simulink model "demo_gs2"  (Simulink 2.20)
settings: Solver=ode45  StartTime=0.0  StopTime=15  MaxStep=0.1  RelTol=1e-3  AbsTol=1e-6
values from neighbouring files (symbols this model uses):
  v = menu('EXACT LINEARIZATION (demo simulations)',    'Exact linearization of SISO system',    'Exact linearization of MIMO system',    'System with unstable zero dynamics')    [demos_exakt.m]    (also in demos_fp.m = menu('PHASE PLANE ANALYSIS (demo simulations)',    '2nd-Orde; demos_gs.m = menu('GAIN SCHEDULING (demo simulations)',    'Input and out)
  x1 = x(j)    [fazrov_auton2.m]
  x2 = x(j+1)    [fazrov_auton2.m]    (also in fazrov_typ1.m = get_param(get_param(gcbh,'Parent'),'UserData'))
undefined symbols (not defined in the file or in its folder): w
libraries: NelinSys x10
settings Model: ConsistencyChecking=off  RTWPlaceOutputsASAP=off

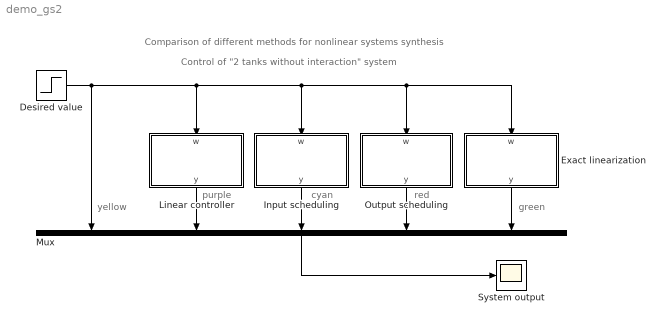
== system demo_gs2 ==
  note: Comparison of different methods for nonlinear systems synthesis
  note: Control of "2 tanks without interaction" system
  note: yellow
  note: purple
  note: cyan
  note: red
  note: green
  Desired value : Step  Time=5  Before=1  After=10
  Exact linearization : Subsystem  Orientation=down
      mask Type: Exact linearization
      mask Display: disp('Exact\nlinearization');
  Input scheduling : Subsystem  Orientation=down
      mask Type: Input scheduling
      mask Display: disp('Input\nscheduling');
  Linear controller : Subsystem  Orientation=down
      mask Type: Linear controller
      mask Display: disp('Linear\ncontroller');
  Mux : Mux  Orientation=down  Inputs=5
  Output scheduling : Subsystem  Orientation=down
      mask Type: Output scheduling
      mask Display: disp('Output\nscheduling');
  System output : Scope
      settings: TickLabels=on  TimeRange=15  YMin=0  YMax=12  SaveToWorkspace=off  SaveName=ScopeData
  wires:
  Output scheduling/1(y) -> Mux/4
  Input scheduling/1(y) -> Mux/3
  Linear controller/1(y) -> Mux/2
  Exact linearization/1(y) -> Mux/5
  Desired value/1 -> Mux/1, Linear controller/1(w), Input scheduling/1(w), Output scheduling/1(w), Exact linearization/1(w)
  Mux/1 -> System output/1

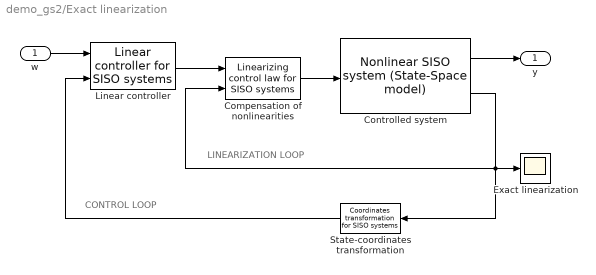
== system demo_gs2/Exact linearization ==
  note: LINEARIZATION LOOP
  note: CONTROL LOOP
  w : Inport  Port=1  PortWidth=-1  SampleTime=-1
  Compensation of nonlinearities : NelinSys/Nonlinear Systems Synthesis/Exact Linearization Blocks/Linearizing control law for SISO systems  n=2  vzorec=x1/sqrt(x2)+2*sqrt(x1)*v  vzorecP=0
  Controlled system : NelinSys/Nonlinear Systems Synthesis/Nonlinear SISO system (State-Space model)  n=2  F=[-sqrt(x1); sqrt(x1)-sqrt(x2)]  Fp=0  G=[1; 0]  Gp=0  H=x2  Hp=0  pp=[0.1; 0.01]
  Exact linearization : Scope
      settings: TickLabels=on  TimeRange=auto  YMin=0  YMax=12  SaveToWorkspace=off  SaveName=ScopeData
  Linear controller : NelinSys/Nonlinear Systems Synthesis/Exact Linearization Blocks/Linear controller for SISO systems  r=2  kor=[-2 -2]  integ=off
  State-coordinates transformation : NelinSys/Nonlinear Systems Synthesis/Exact Linearization Blocks/Coordinates transformation for SISO systems  Orientation=left  n=2  r=2  Z=[x2; sqrt(x1)-sqrt(x2)]  Zp=0
  y : Outport  Port=1
  wires:
  Compensation of nonlinearities/1 -> Controlled system/1
  Linear controller/1 -> Compensation of nonlinearities/1
  State-coordinates transformation/1 -> Linear controller/2
  Controlled system/2 -> State-coordinates transformation/1, Compensation of nonlinearities/2, Exact linearization/1
  w/1 -> Linear controller/1
  Controlled system/1 -> y/1

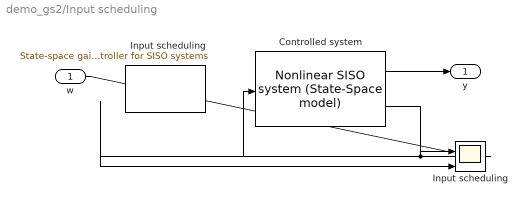
== system demo_gs2/Input scheduling ==
  w : Inport  Port=1  PortWidth=-1  SampleTime=-1
  Controlled system : NelinSys/Nonlinear Systems Synthesis/Nonlinear SISO system (State-Space model)  n=2  F=[-sqrt(x1); sqrt(x1)-sqrt(x2)]  Fp=0  G=[1; 0]  Gp=0  H=x2  Hp=0  pp=[0.1; 0.01]
  Input scheduling : Scope
      settings: TickLabels=on  TimeRange=auto  YMin=0  YMax=12  SaveToWorkspace=off  SaveName=ScopeData
  Input scheduling : NelinSys/Nonlinear Systems Synthesis/Gain Scheduling Blocks/State-space gain-scheduling controller for SISO systems  n=2  vzorec=-(-w^(1/2)+4*w)/w*x1+4*w+1/2*(-w^(1/2)+8*w-16*w^(3/2))/w*(x2-w)  vzorecP=0
  y : Outport  Port=1
  wires:
  Input scheduling/1 -> Controlled system/1
  Controlled system/2 -> Input scheduling/1, Input scheduling/2
  w/1 -> Input scheduling/1
  Controlled system/1 -> y/1

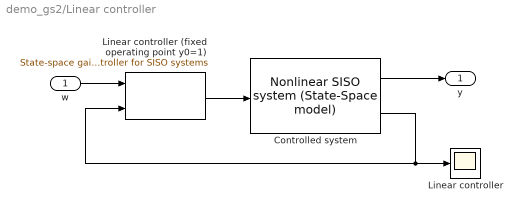
== system demo_gs2/Linear controller ==
  w : Inport  Port=1  PortWidth=-1  SampleTime=-1
  Controlled system : NelinSys/Nonlinear Systems Synthesis/Nonlinear SISO system (State-Space model)  n=2  F=[-sqrt(x1); sqrt(x1)-sqrt(x2)]  Fp=0  G=[1; 0]  Gp=0  H=x2  Hp=0  pp=[0.1; 0.01]
  Linear controller : Scope
      settings: TickLabels=on  TimeRange=auto  YMin=0  YMax=12  SaveToWorkspace=off  SaveName=ScopeData
  Linear controller (fixed operating point y0=1) : NelinSys/Nonlinear Systems Synthesis/Gain Scheduling Blocks/State-space gain-scheduling controller for SISO systems  n=2  vzorec=1/2+8*w-3*x1-9/2*x2  vzorecP=0
  y : Outport  Port=1
  wires:
  Controlled system/1 -> y/1
  w/1 -> Linear controller (fixed operating point y0=1)/1
  Controlled system/2 -> Linear controller (fixed operating point y0=1)/2, Linear controller/1
  Linear controller (fixed operating point y0=1)/1 -> Controlled system/1

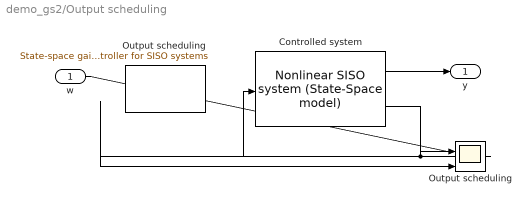
== system demo_gs2/Output scheduling ==
  w : Inport  Port=1  PortWidth=-1  SampleTime=-1
  Controlled system : NelinSys/Nonlinear Systems Synthesis/Nonlinear SISO system (State-Space model)  n=2  F=[-sqrt(x1); sqrt(x1)-sqrt(x2)]  Fp=0  G=[1; 0]  Gp=0  H=x2  Hp=0  pp=[0.1; 0.01]
  Output scheduling : Scope
      settings: TickLabels=on  TimeRange=auto  YMin=0  YMax=12  SaveToWorkspace=off  SaveName=ScopeData
  Output scheduling : NelinSys/Nonlinear Systems Synthesis/Gain Scheduling Blocks/State-space gain-scheduling controller for SISO systems  n=2  vzorec=-(-x2^(1/2)+4*x2)/x2*x1+8*x2^(1/2)*(w-x2)+4*x2  vzorecP=0
  y : Outport  Port=1
  wires:
  Controlled system/1 -> y/1
  w/1 -> Output scheduling/1
  Controlled system/2 -> Output scheduling/2, Output scheduling/1
  Output scheduling/1 -> Controlled system/1
